simulink model "tether001_th"  (R2018b)
settings: Solver=VariableStepAuto  StartTime=0.0  StopTime=0  RelTol=1e-3
values from neighbouring files (symbols this model uses):
  airAngVel = [0 0 0]    [tether001_ts.m]
  airPosVec = [0 0 201]    [tether001_ts.m]
  airVelVec = [0 0 0]    [tether001_ts.m]
  bdy2GndMat = eye(3)    [tether001_ts.m]
  gndAngVel = [0 0 0]    [tether001_ts.m]
  gndPosVec = [0 0 0]    [tether001_ts.m]
  gndVelVec = [0 0 0]    [tether001_ts.m]
  thrReleaseCmd = 0    [tether001_ts.m]
  thrs = OCT.tethers    [tether001_ts.m]
libraries: thrAttachPtKinematics_ul x2, constantUniformFlow_ul x1, tether001_cl x1, winch000_cl x1
settings Model: Creator=mcobb  LastModifiedBy=mcobb

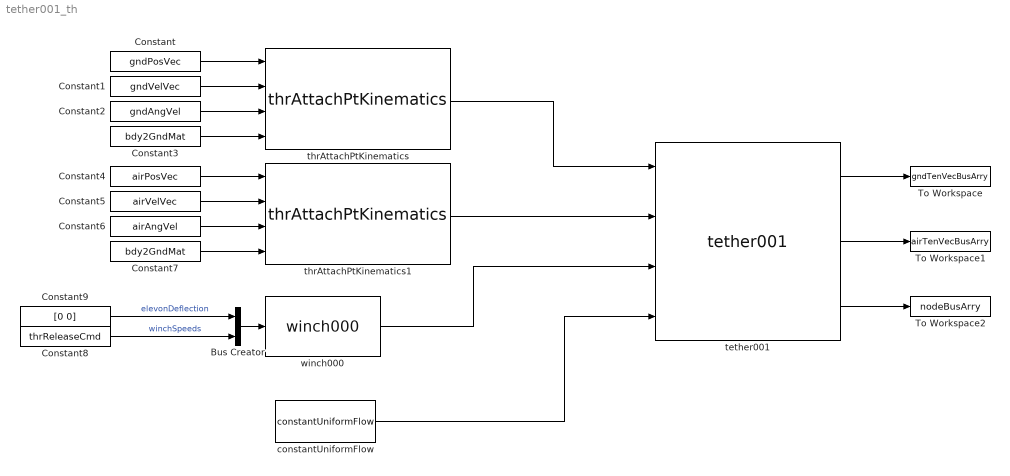
== system tether001_th ==
  Bus Creator : BusCreator  Inputs=2  OutDataTypeStr=Bus: ctrlBus  NonVirtualBus=on
  Constant : Constant  Value=gndPosVec
  Constant1 : Constant  Value=gndVelVec
  Constant2 : Constant  Value=gndAngVel
  Constant3 : Constant  Value=bdy2GndMat
  Constant4 : Constant  Value=airPosVec
  Constant5 : Constant  Value=airVelVec
  Constant6 : Constant  Value=airAngVel
  Constant7 : Constant  Value=bdy2GndMat
  Constant8 : Constant  Value=thrReleaseCmd
  Constant9 : Constant  Value=[0 0]
  To Workspace : ToWorkspace  VariableName=gndTenVecBusArry  SaveFormat=Timeseries  SampleTime=-1
  To Workspace1 : ToWorkspace  VariableName=airTenVecBusArry  SaveFormat=Timeseries  SampleTime=-1
  To Workspace2 : ToWorkspace  VariableName=nodeBusArry  SaveFormat=Timeseries  SampleTime=-1
  constantUniformFlow : constantUniformFlow_ul/constantUniformFlow  SystemSampleTime=-1  VariantControl=VSS_environment_constantUniformFlow
  tether001 : tether001_cl/tether001  LabelModeActiveChoice=NNodeTether  numNodes=thrs.numNodes.Value  tetherStructure=thrs.struct('OCT.tether')  fluidDensity=1000  gravity=9.81
  thrAttachPtKinematics : thrAttachPtKinematics_ul/thrAttachPtKinematics  atchPts=gndMomArm
  thrAttachPtKinematics1 : thrAttachPtKinematics_ul/thrAttachPtKinematics  atchPts=airMomArm
  winch000 : winch000_cl/winch000  SystemSampleTime=-1
  wires:
  winch000/1 -> tether001/3
  constantUniformFlow/1 -> tether001/4
  Constant/1 -> thrAttachPtKinematics/1
  Constant1/1 -> thrAttachPtKinematics/2
  Constant2/1 -> thrAttachPtKinematics/3
  Constant3/1 -> thrAttachPtKinematics/4
  Constant4/1 -> thrAttachPtKinematics1/1
  Constant5/1 -> thrAttachPtKinematics1/2
  Constant6/1 -> thrAttachPtKinematics1/3
  Constant7/1 -> thrAttachPtKinematics1/4
  Constant8/1 -> Bus Creator/2  "winchSpeeds"
  tether001/1 -> To Workspace/1
  tether001/2 -> To Workspace1/1
  tether001/3 -> To Workspace2/1
  Bus Creator/1 -> winch000/1
  Constant9/1 -> Bus Creator/1  "elevonDeflection"
  thrAttachPtKinematics/1 -> tether001/1
  thrAttachPtKinematics1/1 -> tether001/2
